simulink model "Full State Feedback Controller"  (R2025a)
settings: Solver=ode45  StartTime=0.0  StopTime=10  MaxStep=0.001  RelTol=1e-5  AbsTol=1e-6
values from neighbouring files (symbols this model uses):
  A = [0 1 0 0 0 ... (first row only)    [MATHEMATICAL_MODEL.m]
  B = [0 0 ... (first row only)    [MATHEMATICAL_MODEL.m]
  C = [1 0 0 0 0 ... (first row only)    [MATHEMATICAL_MODEL.m]
  D = zeros(5, 2)    [MATHEMATICAL_MODEL.m]
  x0 = [-1; 0; 0; 0; 0]    [MATHEMATICAL_MODEL.m]
settings Model: Creator=User  LastModifiedBy=acer

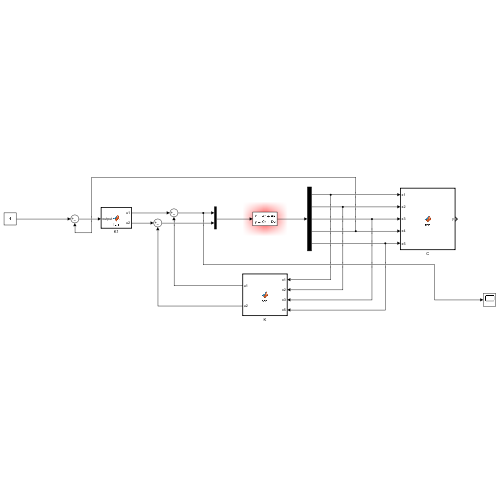
[thumbnail: Simulink's stored preview of the top-level diagram]
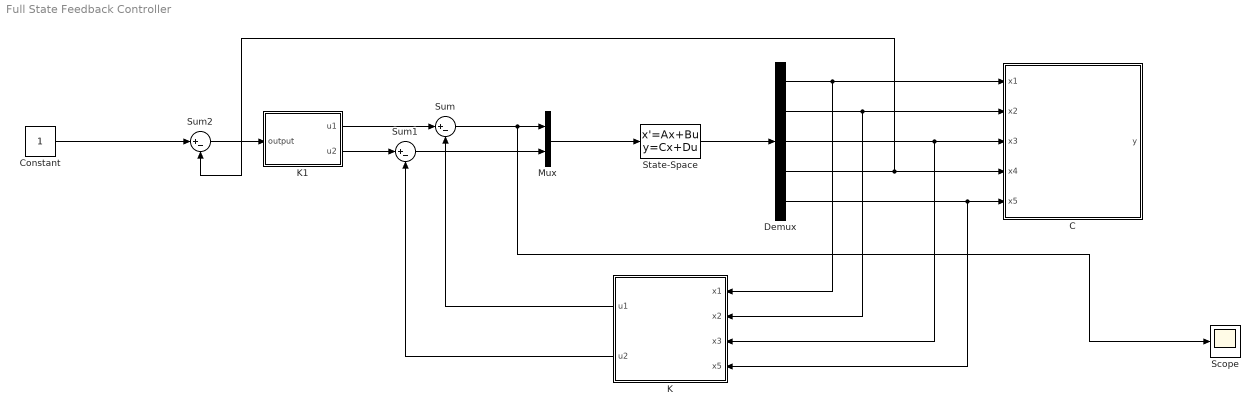
== system Full State Feedback Controller ==
  C : MATLAB Function  TreatAsAtomicUnit=on
  Constant : Constant
  Demux : Demux  Outputs=5
  K : MATLAB Function  TreatAsAtomicUnit=on
  K1 : MATLAB Function  TreatAsAtomicUnit=on
  Mux : Mux  Inputs=2
  Scope : Scope
      settings: ActiveDisplayYMinimum=-1.25266  ActiveDisplayYMaximum=1.27397
  State-Space : StateSpace  A=A  B=B  C=C  D=D  InitialCondition=x0
  Sum : Sum  Inputs=|+-
  Sum1 : Sum  Inputs=|+-
  Sum2 : Sum  Inputs=|+-
  wires:
  Mux/1 -> State-Space/1
  State-Space/1 -> Demux/1
  Sum/1 -> Scope/1, Mux/1
  Sum1/1 -> Mux/2
  K1/1(u1) -> Sum/1
  K1/2(u2) -> Sum1/1
  Demux/1 -> K/1(x1), C/1(x1)
  Demux/2 -> C/2(x2), K/2(x2)
  Demux/3 -> K/3(x3), C/3(x3)
  Demux/5 -> K/4(x5), C/5(x5)
  Demux/4 -> C/4(x4), Sum2/2
  K/2(u2) -> Sum1/2
  K/1(u1) -> Sum/2
  Constant/1 -> Sum2/1
  Sum2/1 -> K1/1(output)

== matlab function Full State Feedback Controller/C ==
  data: x1 input; y output; x2 input; x3 input; x4 input; x5 input
function y = fcn(x1,x2,x3,x4,x5)
X = [x1;x2;x3;x4;x5];
tilt_angle = X(1);
heading_angle=X(4);
y = [tilt_angle;heading_angle];

== matlab function Full State Feedback Controller/K ==
  data: u1 output; u2 output; x1 input; x2 input; x3 input; x5 input
function [u1, u2] = fcn(x1, x2, x3, x5)

    X = [x1; x2; x3; x5];  
    K = [-153.4625 -16.8037  0.7071  1.7307;
         -153.4625 -16.8037  0.7071 -1.7307]; 

    U = K * X; 

    u1 = U(1);  
    u2 = U(2); 
end

== matlab function Full State Feedback Controller/K1 ==
  data: output input; u1 output; u2 output
function [u1, u2] = fcn(output)
              

    K = [2.2361; -2.2361];         

    U = K * output;               

    u1 = U(1);                      
    u2 = U(2);                      
end
